simulink model "ControlsSimulation"  (R2017a)
settings: Solver=VariableStepAuto  StartTime=0.0  StopTime=50  RelTol=1e-3
values from neighbouring files (symbols this model uses):
  ALat = [-0.00695086, -0.25754, -73.9408, 9.81;     -0.894067  , -24.262 , 9.62173 , 0   ;     0.135007   ,  3.12622, -1.51901, 0   ;     0          ,  1      , 0       , 0   ]    [ControlTuning.m]
  ALon = [-0.00958   , 0.0839822 , 0      , -9.81;     -0.266257  , -0.858599 , 73.0863,     0;     0.000153035, -0.0368076, -0.742218,   0;     0          ,          0,         1,   0]    [ControlTuning.m]
  BLat = [Yda/m                    ,                   Ydr/m;          1/zeta*(Iz*Lda + Ixz*Nda), 1/zeta*(Iz*Ldr+Ixz*Ndr);          1/zeta*(Ixz*Lda + Ix*Nda), 1/zeta*(Ixz*Ldr+Ix*Ndr);          0                        , 0                     ]    [ControlTuning.m]
  BLon = [Xde/m, XdT/m; Zde/(m-Zwdot), ZdT/(m-Zwdot) ... (first row only)    [ControlTuning.m]
  KLat = place(ALat,BLat,pdesLat)    [ControlTuning.m]
  KLon = place(ALon,BLon,pdesLon)    [ControlTuning.m]
libraries: simulink x2
settings Model: Creator=alexandermclean  LastModifiedBy=alexandermclean

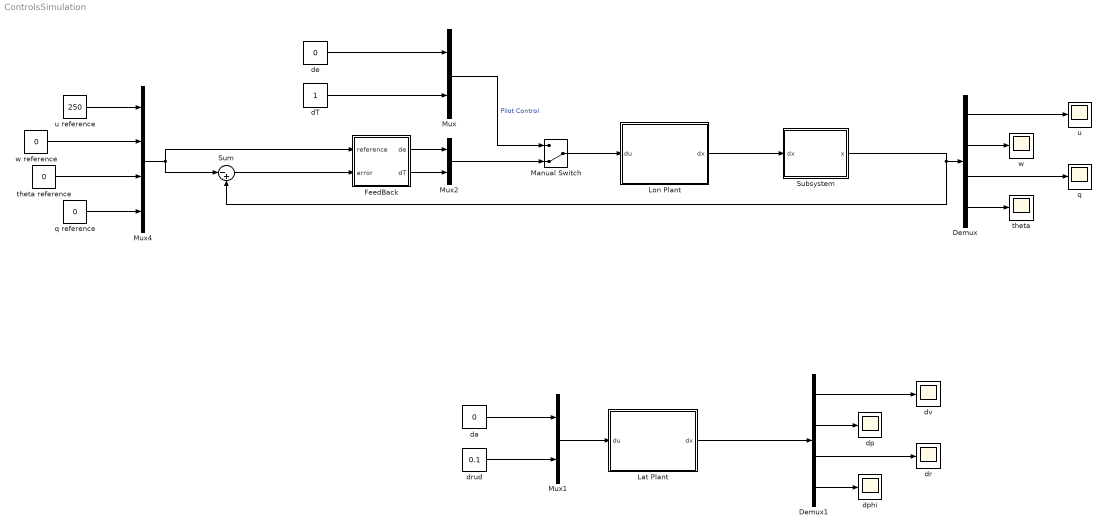
== system ControlsSimulation ==
  " Lon Plant" : Subsystem
  Demux : Demux
  Demux1 : Demux
  FeedBack : Subsystem
  Lat Plant : Subsystem
  Manual Switch : ManualSwitch  CurrentSetting=0
  Mux : Mux  Inputs=2
  Mux1 : Mux  Inputs=2
  Mux2 : Mux  Inputs=2
  Mux4 : Mux
  Subsystem : Subsystem
  Sum : Sum  Inputs=|-+
  dT : Constant
  da : Constant  Value=0
  de : Constant  Value=0
  dp : Scope
  dphi : Scope
  dr : Scope
  drud : Constant  Value=0.1
  dv : Scope
  q : Scope
  q reference : Constant  Value=0
  theta : Scope
  theta reference : Constant  Value=0
  u : Scope
  u reference : Constant  Value=250
  w : Scope
  w reference : Constant  Value=0
  wires:
  Demux/1 -> u/1
  Demux/2 -> w/1
  Demux/3 -> q/1
  Demux/4 -> theta/1
  de/1 -> Mux/1
  dT/1 -> Mux/2
  Mux1/1 -> Lat Plant/1(du)
  da/1 -> Mux1/1
  drud/1 -> Mux1/2
  Lat Plant/1(dx) -> Demux1/1
  Demux1/4 -> dphi/1
  Demux1/3 -> dr/1
  Demux1/1 -> dv/1
  Demux1/2 -> dp/1
  Mux/1 -> Manual Switch/1  "Pilot Control"
  Mux2/1 -> Manual Switch/2
  Manual Switch/1 -> " Lon Plant"/1(du)
  FeedBack/1(de) -> Mux2/1
  FeedBack/2(dT) -> Mux2/2
  theta reference/1 -> Mux4/3
  u reference/1 -> Mux4/1
  w reference/1 -> Mux4/2
  q reference/1 -> Mux4/4
  Mux4/1 -> FeedBack/1(reference), Sum/1
  Sum/1 -> FeedBack/2("error ")
  Subsystem/1(x) -> Sum/2, Demux/1
  " Lon Plant"/1(dx) -> Subsystem/1(dx)

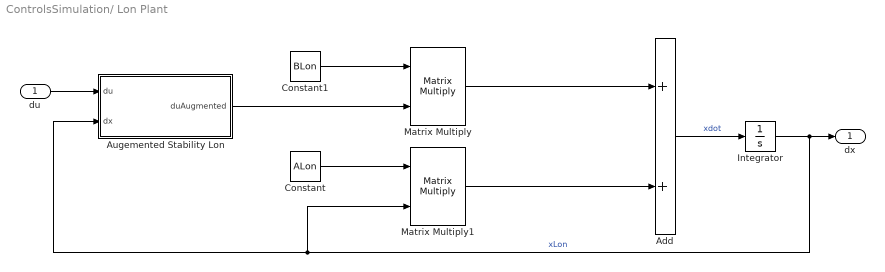
== system ControlsSimulation/ Lon Plant ==
  du : Inport
  Add : Sum
  Augemented Stability Lon : Subsystem
  Constant : Constant  Value=ALon
  Constant1 : Constant  Value=BLon
  Integrator : Integrator
  Matrix Multiply : Product  Multiplication=Matrix(*)
  Matrix Multiply1 : Product  Multiplication=Matrix(*)
  dx : Outport
  wires:
  Constant1/1 -> Matrix Multiply/1
  Matrix Multiply/1 -> Add/1
  Matrix Multiply1/1 -> Add/2
  Constant/1 -> Matrix Multiply1/1
  Add/1 -> Integrator/1  "xdot"
  Integrator/1 -> Matrix Multiply1/2, Augemented Stability Lon/2(dx), dx/1  "xLon"
  du/1 -> Augemented Stability Lon/1(du)
  Augemented Stability Lon/1(duAugmented) -> Matrix Multiply/2

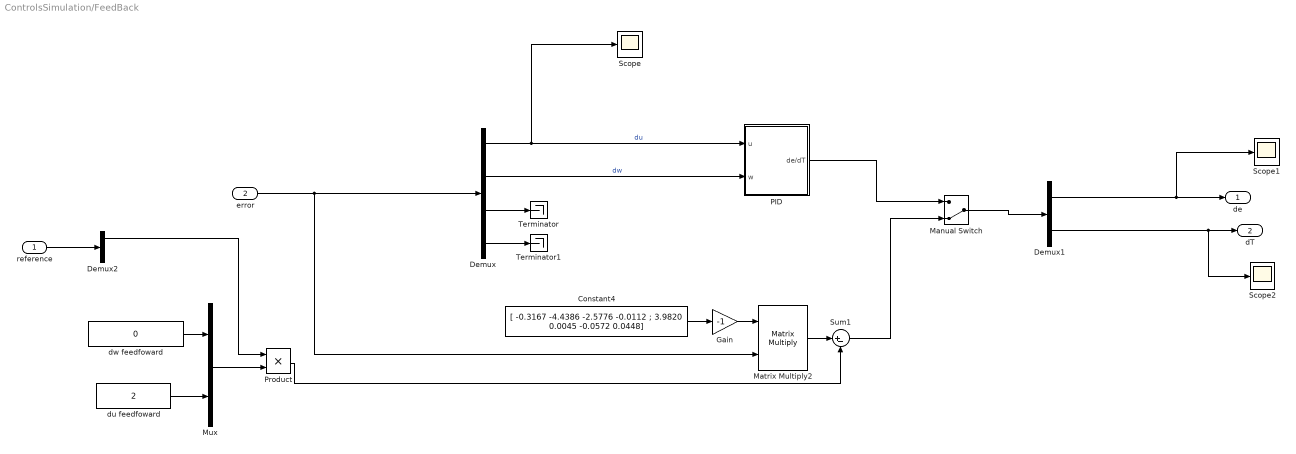
== system ControlsSimulation/FeedBack ==
  reference : Inport
  "error " : Inport  Port=2
  Constant4 : Constant  Value=|
      | [ -0.3167   -4.4386   -2.5776   -0.0112
      | ;  3.9820    0.0045   -0.0572    0.0448]
  Demux : Demux
  Demux1 : Demux  Outputs=2
  Demux2 : Demux  Outputs=2
  Gain : Gain  Gain=-1
  Manual Switch : ManualSwitch  CurrentSetting=0
  Matrix Multiply2 : Product  Multiplication=Matrix(*)
  Mux : Mux  Inputs=2
  PID : Subsystem
  Product : Product
  Scope : Scope
  Scope1 : Scope
  Scope2 : Scope
  Sum1 : Sum  Inputs=|+-
  Terminator : Terminator
  Terminator1 : Terminator
  du feedfoward : Constant  Value=2
  dw feedfoward : Constant  Value=0
  de : Outport
  dT : Outport  Port=2
  wires:
  Demux/3 -> Terminator/1
  Demux/4 -> Terminator1/1
  Demux/1 -> PID/1(u), Scope/1  "du"
  Demux1/2 -> Scope2/1, dT/1
  Demux1/1 -> Scope1/1, de/1
  Demux/2 -> PID/2(w)  "dw"
  Constant4/1 -> Gain/1
  PID/1(de/dT) -> Manual Switch/1
  Manual Switch/1 -> Demux1/1
  Gain/1 -> Matrix Multiply2/1
  Matrix Multiply2/1 -> Sum1/1
  Sum1/1 -> Manual Switch/2
  Mux/1 -> Product/2
  dw feedfoward/1 -> Mux/1
  du feedfoward/1 -> Mux/2
  "error "/1 -> Matrix Multiply2/2, Demux/1
  Product/1 -> Sum1/2
  reference/1 -> Demux2/1
  Demux2/1 -> Product/1

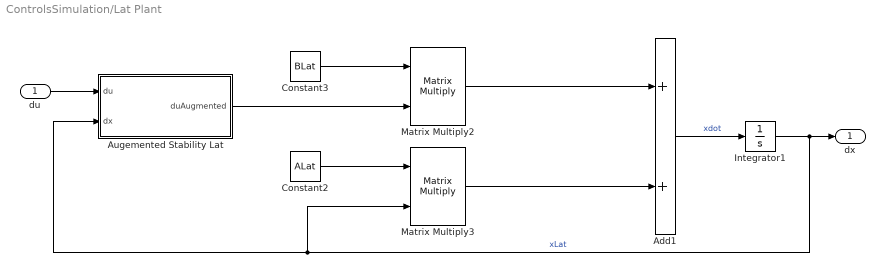
== system ControlsSimulation/Lat Plant ==
  du : Inport
  Add1 : Sum
  Augemented Stability Lat : Subsystem
  Constant2 : Constant  Value=ALat
  Constant3 : Constant  Value=BLat
  Integrator1 : Integrator
  Matrix Multiply2 : Product  Multiplication=Matrix(*)
  Matrix Multiply3 : Product  Multiplication=Matrix(*)
  dx : Outport
  wires:
  Matrix Multiply2/1 -> Add1/1
  Add1/1 -> Integrator1/1  "xdot"
  du/1 -> Augemented Stability Lat/1(du)
  Augemented Stability Lat/1(duAugmented) -> Matrix Multiply2/2
  Constant3/1 -> Matrix Multiply2/1
  Constant2/1 -> Matrix Multiply3/1
  Matrix Multiply3/1 -> Add1/2
  Integrator1/1 -> dx/1, Augemented Stability Lat/2(dx), Matrix Multiply3/2  "xLat"

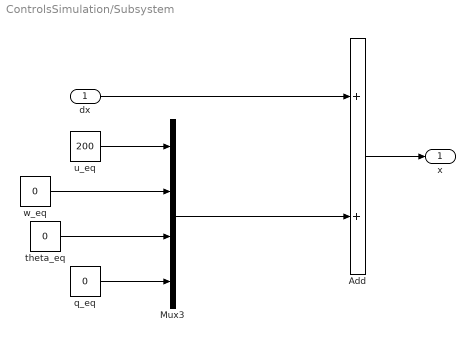
== system ControlsSimulation/Subsystem ==
  dx : Inport
  Add : Sum
  Mux3 : Mux
  q_eq : Constant  Value=0
  theta_eq : Constant  Value=0
  u_eq : Constant  Value=200
  w_eq : Constant  Value=0
  x : Outport
  wires:
  q_eq/1 -> Mux3/4
  u_eq/1 -> Mux3/1
  theta_eq/1 -> Mux3/3
  w_eq/1 -> Mux3/2
  dx/1 -> Add/1
  Mux3/1 -> Add/2
  Add/1 -> x/1

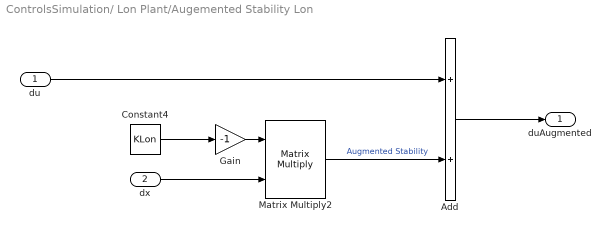
== system ControlsSimulation/ Lon Plant/Augemented Stability Lon ==
  du : Inport
  dx : Inport  Port=2
  Add : Sum
  Constant4 : Constant  Value=KLon
  Gain : Gain  Gain=-1
  Matrix Multiply2 : Product  Multiplication=Matrix(*)
  duAugmented : Outport
  wires:
  Add/1 -> duAugmented/1
  Gain/1 -> Matrix Multiply2/1
  dx/1 -> Matrix Multiply2/2
  Constant4/1 -> Gain/1
  du/1 -> Add/1
  Matrix Multiply2/1 -> Add/2  "Augmented Stability"

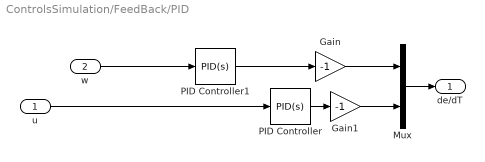
== system ControlsSimulation/FeedBack/PID ==
  u : Inport
  w : Inport  Port=2
  Gain : Gain  Gain=-1
  Gain1 : Gain  Gain=-1
  Mux : Mux  Inputs=2
  PID Controller : simulink/Continuous/PID Controller  Controller=PID  TimeDomain=Continuous-time  SampleTime=-1  IntegratorMethod=Forward Euler  FilterMethod=Forward Euler  Form=Parallel  UseFilter=on  ControllerParametersSource=internal  P=1  I=3  D=2  N=100  InitialConditionSource=internal  InitialConditionForIntegrator=0  InitialConditionForFilter=0  ExternalReset=none  LimitOutput=off  UpperSaturationLimit=inf  LowerSaturationLimit=-inf  LinearizeAsGain=on  AntiWindupMode=none  Kb=1  TrackingMode=off  Kt=1  PParamMin=[]  PParamMax=[]  IParamMin=[]  IParamMax=[]  DParamMin=[]  DParamMax=[]  NParamMin=[]  NParamMax=[]  KbParamMin=[]  KbParamMax=[]  KtParamMin=[]  KtParamMax=[]  POutMin=[]  POutMax=[]  IOutMin=[]  IOutMax=[]  DOutMin=[]  DOutMax=[]  NOutMin=[]  NOutMax=[]  KbOutMin=[]  KbOutMax=[]  KtOutMin=[]  KtOutMax=[]  IntegratorOutMin=[]  IntegratorOutMax=[]  FilterOutMin=[]  FilterOutMax=[]  SumOutMin=[]  SumOutMax=[]  SumI1OutMin=[]  SumI1OutMax=[]  SumI2OutMin=[]  SumI2OutMax=[]  SumI3OutMin=[]  SumI3OutMax=[]  SumDOutMin=[]  SumDOutMax=[]  SaturationOutMin=[]  SaturationOutMax=[]  IntegratorContinuousStateAttributes=''  IntegratorStateMustResolveToSignalObject=off  IntegratorRTWStateStorageClass=Auto  FilterContinuousStateAttributes=''  FilterStateMustResolveToSignalObject=off  FilterRTWStateStorageClass=Auto  DifferentiatorICPrevScaledInput=0  DifferentiatorOutMin=[]  DifferentiatorOutMax=[]  InitialConditionSetting=State (most efficient)
  PID Controller1 : simulink/Continuous/PID Controller  Controller=PID  TimeDomain=Continuous-time  SampleTime=-1  IntegratorMethod=Forward Euler  FilterMethod=Forward Euler  Form=Parallel  UseFilter=on  ControllerParametersSource=internal  P=-1  I=-3  D=-2  N=100  InitialConditionSource=internal  InitialConditionForIntegrator=0  InitialConditionForFilter=0  ExternalReset=none  LimitOutput=off  UpperSaturationLimit=inf  LowerSaturationLimit=-inf  LinearizeAsGain=on  AntiWindupMode=none  Kb=1  TrackingMode=off  Kt=1  PParamMin=[]  PParamMax=[]  IParamMin=[]  IParamMax=[]  DParamMin=[]  DParamMax=[]  NParamMin=[]  NParamMax=[]  KbParamMin=[]  KbParamMax=[]  KtParamMin=[]  KtParamMax=[]  POutMin=[]  POutMax=[]  IOutMin=[]  IOutMax=[]  DOutMin=[]  DOutMax=[]  NOutMin=[]  NOutMax=[]  KbOutMin=[]  KbOutMax=[]  KtOutMin=[]  KtOutMax=[]  IntegratorOutMin=[]  IntegratorOutMax=[]  FilterOutMin=[]  FilterOutMax=[]  SumOutMin=[]  SumOutMax=[]  SumI1OutMin=[]  SumI1OutMax=[]  SumI2OutMin=[]  SumI2OutMax=[]  SumI3OutMin=[]  SumI3OutMax=[]  SumDOutMin=[]  SumDOutMax=[]  SaturationOutMin=[]  SaturationOutMax=[]  IntegratorContinuousStateAttributes=''  IntegratorStateMustResolveToSignalObject=off  IntegratorRTWStateStorageClass=Auto  FilterContinuousStateAttributes=''  FilterStateMustResolveToSignalObject=off  FilterRTWStateStorageClass=Auto  DifferentiatorICPrevScaledInput=0  DifferentiatorOutMin=[]  DifferentiatorOutMax=[]  InitialConditionSetting=State (most efficient)
  de/dT : Outport
  wires:
  w/1 -> PID Controller1/1
  u/1 -> PID Controller/1
  Mux/1 -> de/dT/1
  PID Controller1/1 -> Gain/1
  PID Controller/1 -> Gain1/1
  Gain/1 -> Mux/1
  Gain1/1 -> Mux/2

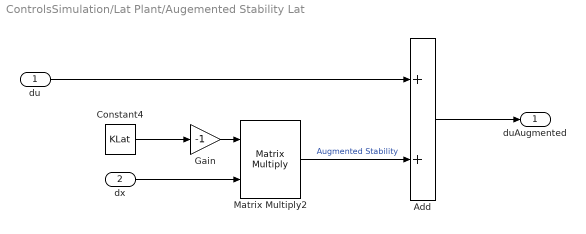
== system ControlsSimulation/Lat Plant/Augemented Stability Lat ==
  du : Inport
  dx : Inport  Port=2
  Add : Sum
  Constant4 : Constant  Value=KLat
  Gain : Gain  Gain=-1
  Matrix Multiply2 : Product  Multiplication=Matrix(*)
  duAugmented : Outport
  wires:
  Matrix Multiply2/1 -> Add/2  "Augmented Stability"
  du/1 -> Add/1
  Constant4/1 -> Gain/1
  dx/1 -> Matrix Multiply2/2
  Gain/1 -> Matrix Multiply2/1
  Add/1 -> duAugmented/1
